simulink model "PID_por_velocidade_por_posicao"  (R2017a)
settings: Solver=VariableStepAuto  StartTime=0.0  StopTime=10.0  RelTol=1e-3
settings Model: Creator=eduardo  LastModifiedBy=eduardo

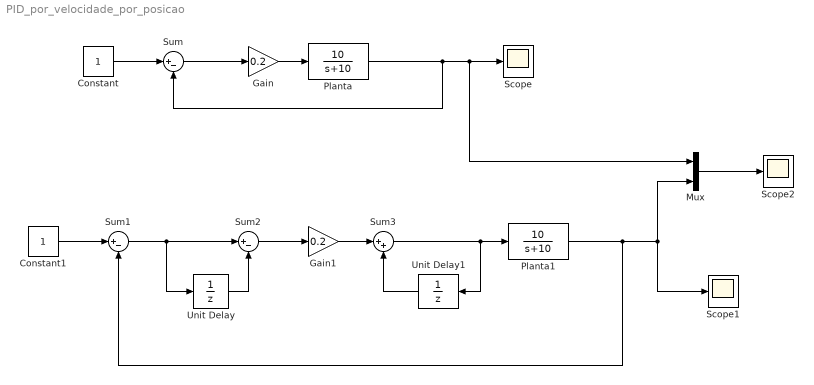
== system PID_por_velocidade_por_posicao ==
  Constant : Constant
  Constant1 : Constant
  Gain : Gain  Gain=0.2
  Gain1 : Gain  Gain=0.2
  Mux : Mux  Inputs=2
  Planta : TransferFcn  Numerator=[10]  Denominator=[1 10]
  Planta1 : TransferFcn  Numerator=[10]  Denominator=[1 10]
  Scope : Scope
  Scope1 : Scope
  Scope2 : Scope
  Sum : Sum  Inputs=|+-
  Sum1 : Sum  Inputs=|+-
  Sum2 : Sum  Inputs=|+-
  Sum3 : Sum  Inputs=|++
  Unit Delay : UnitDelay  SampleTime=-1
  Unit Delay1 : UnitDelay  SampleTime=-1
  wires:
  Constant/1 -> Sum/1
  Gain/1 -> Planta/1
  Sum/1 -> Gain/1
  Planta/1 -> Mux/1, Scope/1, Sum/2
  Planta1/1 -> Sum1/2, Scope1/1, Mux/2
  Constant1/1 -> Sum1/1
  Sum1/1 -> Unit Delay/1, Sum2/1
  Unit Delay/1 -> Sum2/2
  Sum2/1 -> Gain1/1
  Sum3/1 -> Unit Delay1/1, Planta1/1
  Gain1/1 -> Sum3/1
  Unit Delay1/1 -> Sum3/2
  Mux/1 -> Scope2/1
